simulink model "Sys_Ident_AEKmotors"  (R2023a)
settings: Solver=ode3  StartTime=0.0  StopTime=20  RelTol=1e-3  EnableMultiTasking=on
model workspace (MAT data in the model file):
  tickperturn = 1200
libraries: arduinomotorcarrierlib x4, simulink x1
settings Model: ExtModeTrigDuration=2  Creator=auw_a  LastModifiedBy=auw_a
settings SolverCC: AlgebraicLoopSolver=TrustRegion
settings DataIOCC: LimitDataPoints=on  SaveFormat=Array
settings OptimizationCC: ExpressionDepthLimit=2147483647  LifeSpan=Inf  MaxStackSize=64
settings DebuggingCC: UnderspecifiedInitializationDetection=Classic  MergeDetectMultiDrivingBlocksExec=none  FcnCallInpInsideContextMsg=warning  UnconnectedInputMsg=warning  UnconnectedOutputMsg=warning  UnconnectedLineMsg=warning  BusObjectLabelMismatch=error  AllowSymbolicDim=off  StateNameClashWarn=warning  SFUnexpectedBacktrackingDiag=warning  SFNoUnconditionalDefaultTransitionDiag=warning  SFExecutionAtInitializationDiag=none  ArithmeticOperatorsInVariantConditions=warning
settings HardwareCC: ProdBitPerPointer=32  ProdBitPerSizeT=32  ProdBitPerPtrDiffT=32  ProdLargestAtomicInteger=Long  ProdLargestAtomicFloat=Double  ProdWordSize=32  ProdHWDeviceType=ARM Compatible->ARM Cortex
settings ModelReferenceCC: EnableRefExpFcnMdlSchedulingChecks=on  PropagateSignalLabelsOutOfModel=off
settings SFSimCC: SimUseLocalCustomCode=off  CustomCodeUndefinedFunction=UseInterfaceOnly
settings RTWCC: Description=Embedded Coder  SystemTargetFile=ert.tlc  HardwareBoard=Arduino Nano 33 IoT  TemplateMakefile=ert_default_tmf  RTWVerbose=off  RTWUseLocalCustomCode=off  Toolchain=Arduino ARM  BuildConfiguration=Faster Runs
settings CodeAppCC: StateflowObjectComments=on
settings ERTTargetCC: MultiwordLength=2048  ERTCustomFileBanners=off  SupportContinuousTime=on  SupportNonInlinedSFcns=on  RemoveResetFunc=off  SupportVariableSizeSignals=on  ModelStepFunctionPrototypeControlCompliant=off  ExtModeTransport=3  ExtModeStaticAlloc=on  ExtModeAutomaticAllocSize=off  ExtModeStaticAllocSize=8192  ExtModeMexFile=ext_xcp  ExtModeIntrfLevel=Level2 - Open  ConvertIfToSwitch=off  SuppressUnreachableDefaultCases=off
settings ConfigComp: CovMetricSettings=dw  CovSaveCumulativeToWorkspaceVar=on  CovSaveSingleToWorkspaceVar=on  CovExternalEMLEnable=off  CovSFcnEnable=off

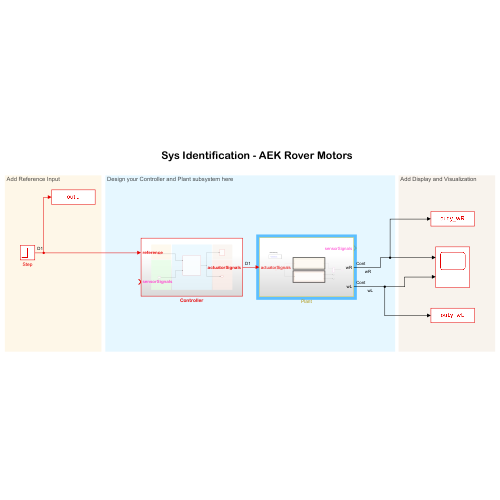
[thumbnail: Simulink's stored preview of the top-level diagram]
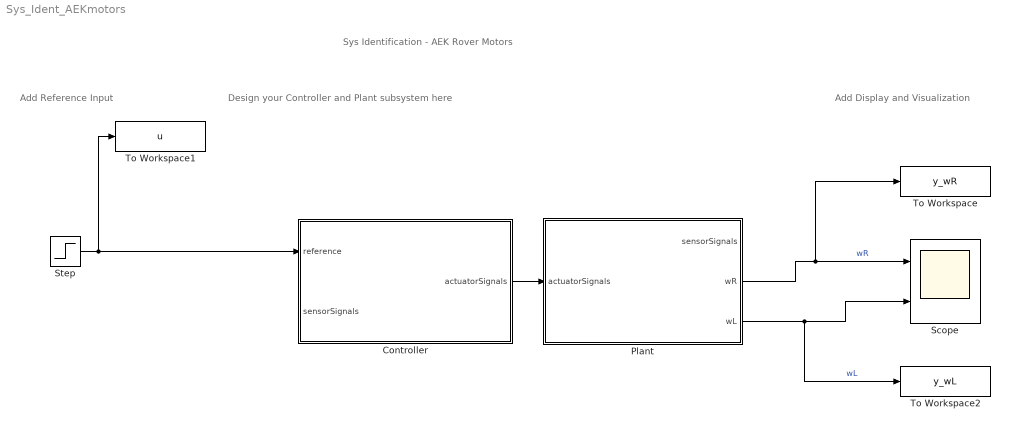
== system Sys_Ident_AEKmotors ==
  note: Sys Identification - AEK Rover Motors
  note: Add Display and Visualization
  note: Add Reference Input
  note: Design your Controller and Plant subsystem here
  Controller : Subsystem
  Plant : Subsystem
  Scope : Scope  NumInputPorts=2
  Step : Step  After=20  SampleTime=0.01
  To Workspace : ToWorkspace  VariableName=y_wR  SampleTime=-1
      settings: Save2DSignal=2-D array (concatenate along first dimension)
  To Workspace1 : ToWorkspace  VariableName=u  SampleTime=-1
      settings: Save2DSignal=2-D array (concatenate along first dimension)
  To Workspace2 : ToWorkspace  VariableName=y_wL  SampleTime=-1
      settings: Save2DSignal=2-D array (concatenate along first dimension)
  wires:
  Step/1 -> Controller/1(reference), To Workspace1/1
  Controller/1(actuatorSignals) -> Plant/1(actuatorSignals)
  Plant/2(wR) -> To Workspace/1, Scope/1  "wR"
  Plant/3(wL) -> To Workspace2/1, Scope/2  "wL"

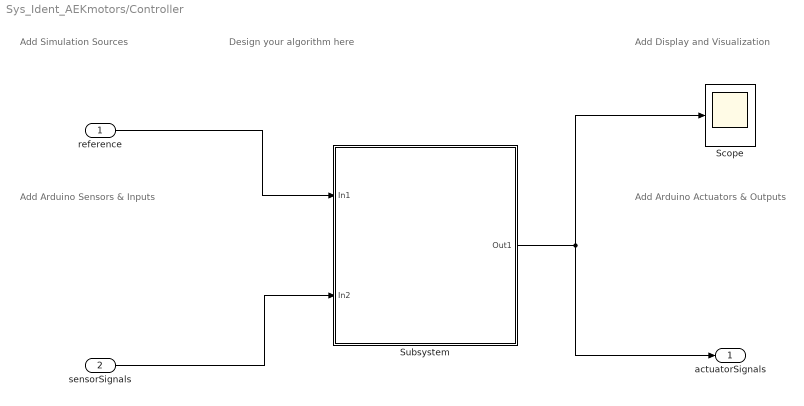
== system Sys_Ident_AEKmotors/Controller ==
  note: Add Display and Visualization
  note: Add Arduino Sensors & Inputs
  note: Design your algorithm here
  note: Add Simulation Sources
  note: Add Arduino Actuators & Outputs
  reference : Inport
  sensorSignals : Inport  Port=2
  Scope : Scope
  Subsystem : Subsystem
  actuatorSignals : Outport  VectorParamsAs1DForOutWhenUnconnected=off
  wires:
  sensorSignals/1 -> Subsystem/2(In2)
  reference/1 -> Subsystem/1(In1)
  Subsystem/1(Out1) -> actuatorSignals/1, Scope/1

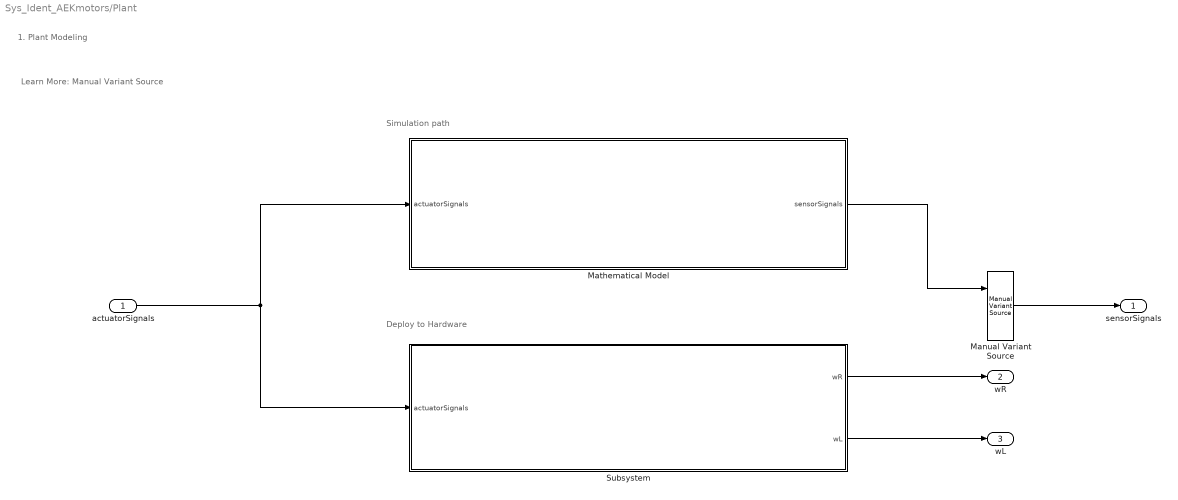
== system Sys_Ident_AEKmotors/Plant ==
  note: Deploy to Hardware
  note: Simulation path
  note: Learn More:
      |
      | Manual Variant Source
  note: 1. Plant Modeling
  actuatorSignals : Inport
  Manual Variant Source : simulink/Signal Routing/Manual Variant Source  NumChoices=2  LabelModeActiveChoice=V_2
  Mathematical Model : Subsystem  VariantControl=plantModel==1
  Subsystem : Subsystem  VariantControl=plantModel==2
  sensorSignals : Outport  VectorParamsAs1DForOutWhenUnconnected=off
  wR : Outport  Port=2  VectorParamsAs1DForOutWhenUnconnected=off
  wL : Outport  Port=3  VectorParamsAs1DForOutWhenUnconnected=off
  wires:
  actuatorSignals/1 -> Mathematical Model/1(actuatorSignals), Subsystem/1(actuatorSignals)
  Mathematical Model/1(sensorSignals) -> Manual Variant Source/1
  Manual Variant Source/1 -> sensorSignals/1
  Subsystem/1(wR) -> wR/1
  Subsystem/2(wL) -> wL/1

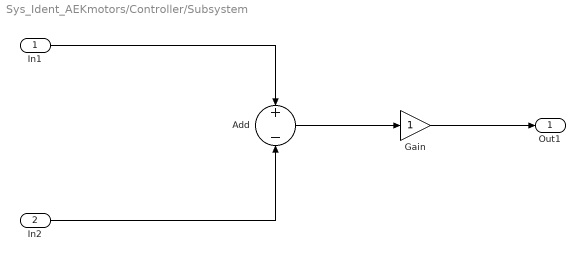
== system Sys_Ident_AEKmotors/Controller/Subsystem ==
  In1 : Inport
  In2 : Inport  Port=2
  Add : Sum  Inputs=+-
  Gain : Gain
  Out1 : Outport  VectorParamsAs1DForOutWhenUnconnected=off
  wires:
  In2/1 -> Add/2
  In1/1 -> Add/1
  Add/1 -> Gain/1
  Gain/1 -> Out1/1

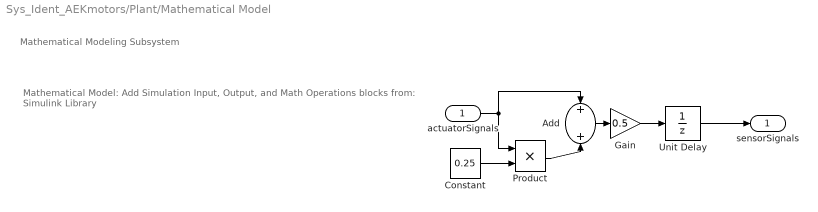
== system Sys_Ident_AEKmotors/Plant/Mathematical Model ==
  note: Mathematical Model:
      |
      | Add Simulation Input, Output, and Math Operations blocks from:
      | Simulink Library
  note: Mathematical Modeling Subsystem
  actuatorSignals : Inport
  Add : Sum
  Constant : Constant  Value=0.25  SampleTime=-1
  Gain : Gain  Gain=0.5
  Product : Product
  Unit Delay : UnitDelay  SampleTime=-1  HasFrameUpgradeWarning=on
  sensorSignals : Outport  VectorParamsAs1DForOutWhenUnconnected=off
  wires:
  actuatorSignals/1 -> Product/1, Add/1
  Add/1 -> Gain/1
  Product/1 -> Add/2
  Gain/1 -> Unit Delay/1
  Constant/1 -> Product/2
  Unit Delay/1 -> sensorSignals/1

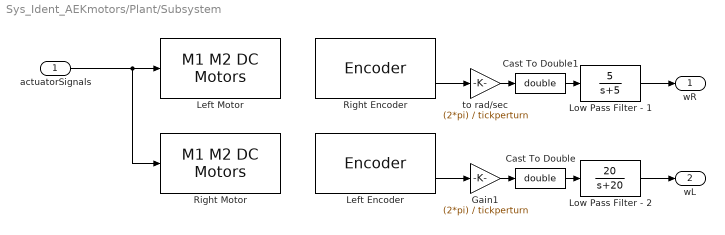
== system Sys_Ident_AEKmotors/Plant/Subsystem ==
  actuatorSignals : Inport
  Cast To Double : DataTypeConversion  OutDataTypeStr=double  SaturateOnIntegerOverflow=off  RndMeth=Floor
  Cast To Double1 : DataTypeConversion  OutDataTypeStr=double  SaturateOnIntegerOverflow=off  RndMeth=Floor
  Gain1 : Gain  Gain=(2*pi) / tickperturn
  Left Encoder : arduinomotorcarrierlib/Encoder  SlaveAddress=uint8( hex2dec( '66' ) )  blockPlatform=ARDUINO  Encoder=2  ShowSpeed=on  ResetOption=on  SampleTime=0.01
  Left Motor : arduinomotorcarrierlib/M1 M2 DC Motors  SlaveAddress=uint8( hex2dec( '66' ) )  blockPlatform=ARDUINO  MotorNumber=M2  MotorCarrierPWMFreq=100
  Low Pass Filter - 1 : TransferFcn  Numerator=[5]  Denominator=[1 5]
  Low Pass Filter - 2 : TransferFcn  Numerator=[20]  Denominator=[1 20]
  Right Encoder : arduinomotorcarrierlib/Encoder  SlaveAddress=uint8( hex2dec( '66' ) )  blockPlatform=ARDUINO  Encoder=1  ShowSpeed=on  ResetOption=on  SampleTime=0.01
  Right Motor : arduinomotorcarrierlib/M1 M2 DC Motors  SlaveAddress=uint8( hex2dec( '66' ) )  blockPlatform=ARDUINO  MotorNumber=M1  MotorCarrierPWMFreq=100
  to rad/sec : Gain  Gain=(2*pi) / tickperturn
  wR : Outport  VectorParamsAs1DForOutWhenUnconnected=off
  wL : Outport  Port=2  VectorParamsAs1DForOutWhenUnconnected=off
  wires:
  actuatorSignals/1 -> Right Motor/1, Left Motor/1
  Right Encoder/2 -> to rad/sec/1
  Left Encoder/2 -> Gain1/1
  Low Pass Filter - 1/1 -> wR/1
  Low Pass Filter - 2/1 -> wL/1
  Gain1/1 -> Cast To Double/1
  Cast To Double/1 -> Low Pass Filter - 2/1
  to rad/sec/1 -> Cast To Double1/1
  Cast To Double1/1 -> Low Pass Filter - 1/1
